simulink model "Heli_inner_loop"  (R2018b)
settings: Solver=FixedStepDiscrete  StartTime=0.0  StopTime=10.0  FixedStep=0.01  RelTol=1e-3  EnableMultiTasking=on
libraries: HeliLibrary x3, simulink x1
Description:
  | This model implements a multi-variable inner loop control for a helicopter.  The control loop stabilizes the pitch rate, roll rate and yaw rate of the helicopter.
settings Model: Creator=bpotter  LastModifiedBy=bpotter
settings DataIOCC: LimitDataPoints=on  SaveFormat=Array
settings OptimizationCC: BlockReduction=off  DefaultParameterBehavior=Inlined  UseDivisionForNetSlopeComputation=on  PassReuseOutputArgsAs=Individual arguments  InitFltsAndDblsToZero=on  EfficientFloat2IntCast=on  EfficientMapNaN2IntZero=off  LifeSpan=inf  MaxStackSize=inf
settings DebuggingCC: SignalInfNanChecking=error  SignalRangeChecking=error  ReadBeforeWriteMsg=EnableAllAsError  WriteAfterWriteMsg=EnableAllAsError  WriteAfterReadMsg=EnableAllAsError  AlgebraicLoopMsg=error  ArtificialAlgebraicLoopMsg=error  SaveWithDisabledLinksMsg=error  SaveWithParameterizedLinksMsg=error  BlockPriorityViolationMsg=error  SolverPrmCheckMsg=error  InheritedTsInSrcMsg=error  SingleTaskRateTransMsg=error  TasksWithSamePriorityMsg=error  SigSpecEnsureSampleTimeMsg=error  CheckMatrixSingularityMsg=error  IntegerOverflowMsg=error  ParameterUnderflowMsg=error  ParameterPrecisionLossMsg=error  ParameterTunabilityLossMsg=error  UnderSpecifiedDataTypeMsg=error  UnnecessaryDatatypeConvMsg=warning  VectorMatrixConversionMsg=error  SignalLabelMismatchMsg=error  UnconnectedInputMsg=error  UnconnectedOutputMsg=error  UnconnectedLineMsg=error  SFcnCompatibilityMsg=error  UniqueDataStoreMsg=error  BusObjectLabelMismatch=error  RootOutportRequireBusObject=error  AssertControl=DisableAll  AllowSymbolicDim=off  ModelReferenceIOMsg=error  ModelReferenceIOMismatchMessage=error  UnknownTsInhSupMsg=error  ModelReferenceDataLoggingMessage=error  StateNameClashWarn=warning  LibraryContextMissingDiagnostic=none  StrictBusMsg=ErrorOnBusTreatedAsVector  NonBusSignalsTreatedAsBus=error  SFInvalidInputDataAccessInChartInitDiag=error  SFTransitionOutsideNaturalParentDiag=error  SFUnreachableExecutionPathDiag=error  SFUndirectedBroadcastEventsDiag=error  SFTransitionActionBeforeConditionDiag=error  SFExecutionAtInitializationDiag=none  IntegerSaturationMsg=error
settings HardwareCC: ProdBitPerPointer=32  ProdBitPerSizeT=32  ProdBitPerPtrDiffT=32  ProdWordSize=32  ProdHWDeviceType=Intel->x86-32 (Windows32)  TargetIntDivRoundTo=Zero
settings ModelReferenceCC: PropagateSignalLabelsOutOfModel=off
settings SFSimCC: SimUseLocalCustomCode=off  CompileTimeRecursionLimit=0  EnableRuntimeRecursion=off  MATLABDynamicMemAlloc=off
settings RTWCC: SystemTargetFile=ert.tlc  TemplateMakefile=ert_default_tmf  GenerateReport=on  RTWUseLocalCustomCode=off  IncludeHyperlinkInReport=on  LaunchReport=on  PortableWordSizes=on  GenerateTraceInfo=on  GenerateTraceReport=on  GenerateTraceReportSl=on  GenerateTraceReportSf=on  GenerateTraceReportEml=on
settings CodeAppCC: ForceParamTrailComments=on  IgnoreCustomStorageClasses=off  MangleLength=4  StateflowObjectComments=on  ReqsInCode=on
settings ERTTargetCC: TargetLangStandard=C99 (ISO)  UtilityFuncGeneration=Shared location  MultiwordLength=2048  GenerateSampleERTMain=on  IncludeMdlTerminateFcn=off  SuppressErrorStatus=on  SupportAbsoluteTime=off  SupportNonFinite=off  ParenthesesLevel=Maximum  CastingMode=Standards  GenerateSharedConstants=off  ERTCustomFileTemplate=example_file_process.tlc  ERTFilePackagingFormat=Compact  PreserveExpressionOrder=on  PreserveIfCondition=on  ConvertIfToSwitch=off  SuppressUnreachableDefaultCases=off  EnableSignedLeftShifts=off  EnableSignedRightShifts=off
settings ConfigComp: CovMetricSettings=dw  CovHtmlReporting=on  CovSaveCumulativeToWorkspaceVar=on  CovSaveSingleToWorkspaceVar=on  CovExternalEMLEnable=off  CovSFcnEnable=off  PSVerificationMode=BugFinder  PSResultDir=BugFinder_results_$ModelName$  PSAutoStubLUT=off

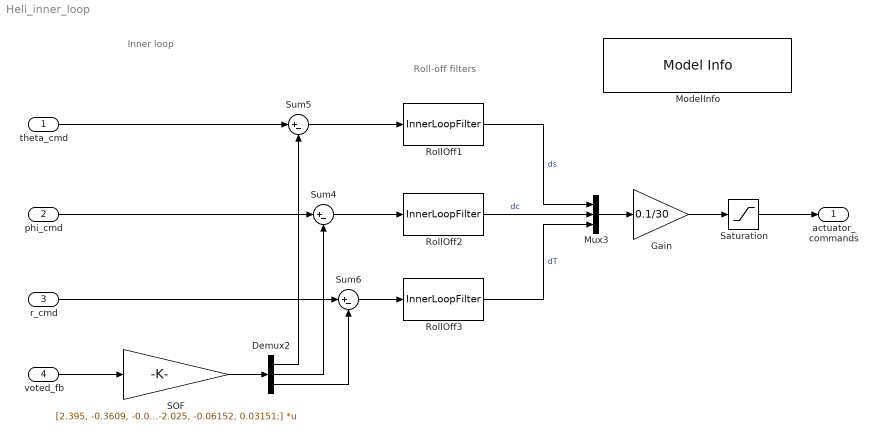
== system Heli_inner_loop ==
  note: Roll-off filters
  note: Inner loop
  theta_cmd : Inport  RequirementInfo={} %GIDa_651dd069_3e46_4718_8fbf_45e69644669e  OutMin=-30  OutMax=30  OutDataTypeStr=double  PortDimensions=1  SampleTime=0.01
  phi_cmd : Inport  RequirementInfo={} %GIDa_7d4fd3b3_16ea_42ea_bc7f_1135a5c98576  Port=2  OutMin=-30  OutMax=30  OutDataTypeStr=double  PortDimensions=1  SampleTime=0.01
  r_cmd : Inport  RequirementInfo={} %GIDa_83c549e4_3c18_44e9_bdac_2c7a7d1b17ce  Port=3  OutMin=-30  OutMax=30  OutDataTypeStr=double  PortDimensions=1  SampleTime=0.01
  voted_fb : Inport  RequirementInfo={} %GIDa_0d5297d6_8cea_45cd_aede_4ebda2178ef9  Port=4  OutMin=-180  OutMax=180  OutDataTypeStr=double  PortDimensions=5  SampleTime=0.01
  Demux2 : Demux  RequirementInfo={} %GIDa_235c591a_aa73_491a_a9e4_dc069ef42454  Outputs=3
  Gain : Gain  RequirementInfo={} %GIDa_f1559598_2cf4_432b_b97f_9921cd96ff54  Gain=0.1/30
  ModelInfo : simulink/Model-Wide Utilities/Model Info  Frame=on  DisplayStringWithTags=|  HorizontalTextAlignment=Center  LeftAlignmentValue=0.5
      | Model Name: %<ModelName>
      | Model Version: %<ModelVersion>
      | Last Modified: %<LastModificationDate>
      | 
      | Copyright 2016 The MathWorks, Inc.
  Mux3 : Mux  RequirementInfo={} %GIDa_84a5a0ba_ecf5_44fe_b1b6_a5620a3d86f2  Inputs=3
  RollOff1 : HeliLibrary/InnerLoopFilter  Tag=FilterWizardSubSystem  RequirementInfo={} %GIDa_ac7f675d_0c04_474f_b6aa_16ea1999b46b  SystemSampleTime=-1
      settings: AttributesFormatString=@100Hz
  RollOff2 : HeliLibrary/InnerLoopFilter  Tag=FilterWizardSubSystem  RequirementInfo={} %GIDa_350d2289_ad89_4b99_9e80_fa521099ee91  SystemSampleTime=-1
      settings: AttributesFormatString=@100Hz
  RollOff3 : HeliLibrary/InnerLoopFilter  Tag=FilterWizardSubSystem  RequirementInfo={} %GIDa_6b9b405b_82fc_4a51_bdc3_80ac9659e3ea  SystemSampleTime=-1
      settings: AttributesFormatString=@100Hz
  SOF : Gain  RequirementInfo={} %GIDa_7f751ee0_858c_4337_95eb_77b3a727b4db  Gain=[2.395, -0.3609, -0.002145, 0.8087, -0.0205; -0.1427, -1.115, 0.04573, -0.04318, -0.1007; -0.02792, -0.02229, -2.025, -0.06152, 0.03151;]  Multiplication=Matrix(K*u) (u vector)
  Saturation : Saturate  UpperLimit=0.1  LowerLimit=-0.1
  Sum4 : Sum  RequirementInfo={} %GIDa_7718e79a_1f37_4b40_8c1f_a001102bf4cd  Inputs=|+-
  Sum5 : Sum  RequirementInfo={} %GIDa_1a76d1b0_44cf_4b26_8d87_94f41ef1f3b5  Inputs=|+-
  Sum6 : Sum  RequirementInfo={} %GIDa_71156066_b5f6_44b8_bfcd_31ab60b0f053  Inputs=|+-
  actuator_commands : Outport  RequirementInfo={} %GIDa_7aee70b8_1e0c_4ab4_a128_8f534750b0ce
  wires:
  Mux3/1 -> Gain/1
  Sum4/1 -> RollOff2/1
  RollOff3/1 -> Mux3/3  "dT"
  RollOff2/1 -> Mux3/2  "dc"
  RollOff1/1 -> Mux3/1  "ds"
  theta_cmd/1 -> Sum5/1
  Sum5/1 -> RollOff1/1
  SOF/1 -> Demux2/1
  phi_cmd/1 -> Sum4/1
  r_cmd/1 -> Sum6/1
  Sum6/1 -> RollOff3/1
  Demux2/1 -> Sum5/2
  Demux2/2 -> Sum4/2
  Demux2/3 -> Sum6/2
  voted_fb/1 -> SOF/1
  Gain/1 -> Saturation/1
  Saturation/1 -> actuator_commands/1
